simulink library "lib_cartesian_controllers"  (Simulink 9.0)
settings: Solver=ode45  StartTime=0.0  StopTime=10.0  RelTol=1e-3  EnableMultiTasking=on
undefined symbols (not defined in the file): k_D_p, k_D_r, k_p, k_P_p, k_P_r, k_r, k_t
libraries: lib_cartesian_controllers x10, lib_transformations x4
settings Model: SuppressorTable=22 serialization::archive 11 0 6 0 0 0 11 0  Creator=schappler  LastModifiedBy=schappler

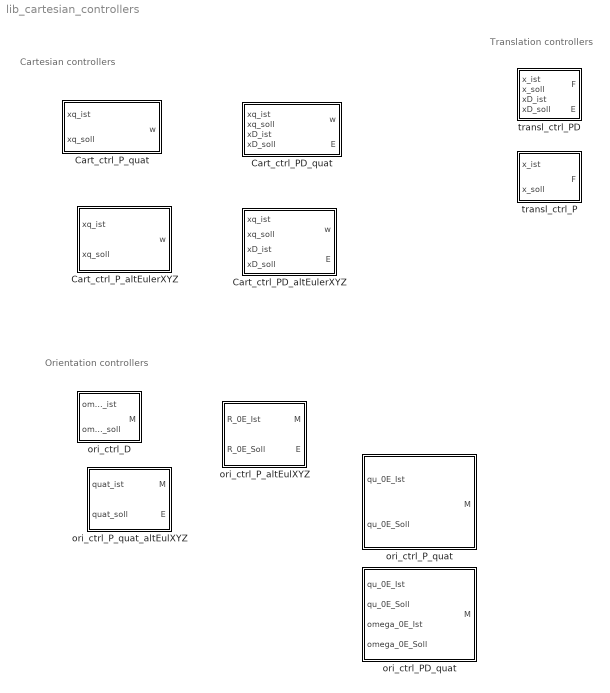
== system lib_cartesian_controllers ==
  note: Cartesian controllers
  note: Translation controllers
  note: Orientation controllers
  Cart_ctrl_PD_altEulerXYZ : Subsystem  mask{k_P_p=k_P_p, k_P_r=k_P_r, k_D_p=k_D_p, k_D_r=k_D_r}
      mask prompts: k_P_p "Translatorische Steifigkeit"; k_P_r "Rotatorische Steifigkeit"; k_D_p "Translatorische Dämpfung"; k_D_r "Rotatorische Dämpfung"
  Cart_ctrl_PD_quat : Subsystem  mask{k_P_p=k_P_p, k_P_r=k_P_r, k_D_p=k_D_p, k_D_r=k_D_r}
      mask prompts: k_P_p "Translatorische Steifigkeit"; k_P_r "Rotatorische Steifigkeit"; k_D_p "Translatorische Dämpfung"; k_D_r "Rotatorische Dämpfung"
  Cart_ctrl_P_altEulerXYZ : Subsystem  mask{k_p=k_p, k_r=k_r}
      mask prompts: k_p "Positions-Verstärkung (Steifigkeit)"; k_r "Rotations-Verstärkung (Drehsteifigkeit)"
  Cart_ctrl_P_quat : Subsystem  mask{k_t=k_t, k_r=k_r}
      mask prompts: k_t "Translatorische Steifigkeit"; k_r "Rotatorische Steifigkeit"
  ori_ctrl_D : Subsystem  mask{k=k_r}
      mask prompts: k "Proportionalverstärkung"
  ori_ctrl_PD_quat : Subsystem  mask{k_P_r=k_P_r, k_D_r=k_D_r}
      mask prompts: k_P_r "Rotatorische Steifigkeit"; k_D_r "Rotatorische Dämpfung"
  ori_ctrl_P_altEulXYZ : Subsystem  mask{k=k_r}
      mask prompts: k "Proportionalverstärkung"
  ori_ctrl_P_quat : Subsystem  mask{k_P_r=k_P_r}
      mask prompts: k_P_r "Rotatorische Steifigkeit"
  ori_ctrl_P_quat_altEulXYZ : Subsystem  mask{k_P_r=k_P_r}
      mask prompts: k_P_r "Rotatorische Steifigkeit"
  transl_ctrl_P : Subsystem  mask{k=k_t}
      mask prompts: k "Proportionalverstärkung"
  transl_ctrl_PD : Subsystem  mask{k_P_p=k_P_p, k_D_p=k_D_p}
      mask prompts: k_P_p "Proportionalverstärkung (k_P_p)"; k_D_p "Differentialverstärkung k_D_p"

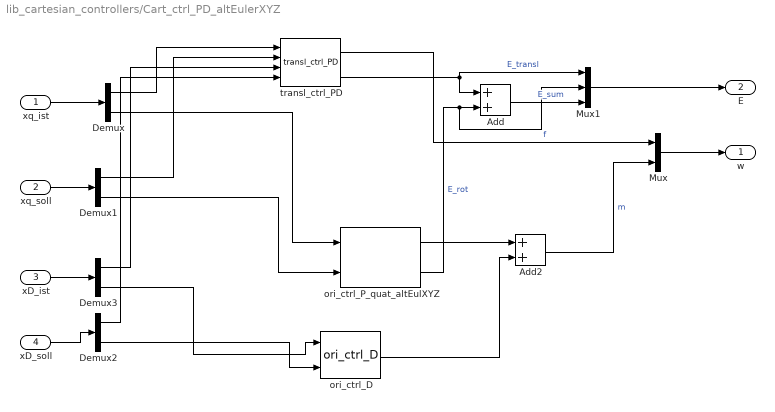
== system lib_cartesian_controllers/Cart_ctrl_PD_altEulerXYZ ==
  xq_ist : Inport  PortDimensions=7
  xq_soll : Inport  Port=2  PortDimensions=7
  xD_ist : Inport  Port=3  PortDimensions=6
  xD_soll : Inport  Port=4  PortDimensions=6
  Add : Sum
  Add2 : Sum
  Demux : Demux  Outputs=[3 4]
  Demux1 : Demux  Outputs=[3 4]
  Demux2 : Demux  Outputs=[3 3]
  Demux3 : Demux  Outputs=[3 3]
  Mux : Mux  Inputs=[3 3]
  Mux1 : Mux  Inputs=[1 1 1]
  ori_ctrl_D : lib_cartesian_controllers/ori_ctrl_D  k=k_D_r
  ori_ctrl_P_quat_altEulXYZ : lib_cartesian_controllers/ori_ctrl_P_quat_altEulXYZ  k_P_r=k_P_r
  transl_ctrl_PD : lib_cartesian_controllers/transl_ctrl_PD  k_P_p=k_P_p  k_D_p=k_D_p
  w : Outport
  E : Outport  Port=2
  wires:
  transl_ctrl_PD/1 -> Mux/1  "f"
  ori_ctrl_P_quat_altEulXYZ/1 -> Add2/1
  Demux1/1 -> transl_ctrl_PD/2
  xq_soll/1 -> Demux1/1
  Demux/1 -> transl_ctrl_PD/1
  xq_ist/1 -> Demux/1
  Demux/2 -> ori_ctrl_P_quat_altEulXYZ/1
  Demux1/2 -> ori_ctrl_P_quat_altEulXYZ/2
  xD_soll/1 -> Demux2/1
  xD_ist/1 -> Demux3/1
  Demux3/1 -> transl_ctrl_PD/3
  Demux2/1 -> transl_ctrl_PD/4
  Demux3/2 -> ori_ctrl_D/1
  Demux2/2 -> ori_ctrl_D/2
  ori_ctrl_D/1 -> Add2/2
  Mux/1 -> w/1
  Add2/1 -> Mux/2  "m"
  transl_ctrl_PD/2 -> Add/1, Mux1/1  "E_transl"
  ori_ctrl_P_quat_altEulXYZ/2 -> Mux1/2, Add/2  "E_rot"
  Mux1/1 -> E/1
  Add/1 -> Mux1/3  "E_sum"

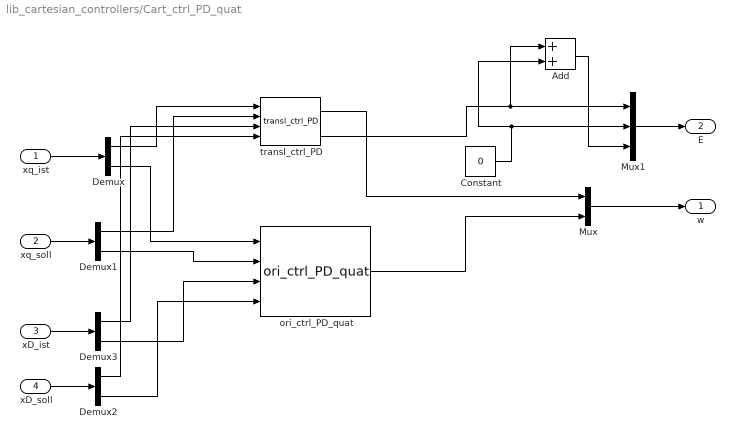
== system lib_cartesian_controllers/Cart_ctrl_PD_quat ==
  xq_ist : Inport  PortDimensions=7
  xq_soll : Inport  Port=2  PortDimensions=7
  xD_ist : Inport  Port=3  PortDimensions=6
  xD_soll : Inport  Port=4  PortDimensions=6
  Add : Sum
  Constant : Constant  Value=0
  Demux : Demux  Outputs=[3 4]
  Demux1 : Demux  Outputs=[3 4]
  Demux2 : Demux  Outputs=[3 3]
  Demux3 : Demux  Outputs=[3 3]
  Mux : Mux  Inputs=[3 3]
  Mux1 : Mux  Inputs=[1 1 1]
  ori_ctrl_PD_quat : lib_cartesian_controllers/ori_ctrl_PD_quat  k_P_r=k_P_r  k_D_r=k_D_r
  transl_ctrl_PD : lib_cartesian_controllers/transl_ctrl_PD  k_P_p=k_P_p  k_D_p=k_D_p
  w : Outport
  E : Outport  Port=2
  wires:
  Demux1/1 -> transl_ctrl_PD/2
  xq_soll/1 -> Demux1/1
  Demux/1 -> transl_ctrl_PD/1
  xq_ist/1 -> Demux/1
  Demux/2 -> ori_ctrl_PD_quat/1
  Demux1/2 -> ori_ctrl_PD_quat/2
  transl_ctrl_PD/1 -> Mux/1
  xD_soll/1 -> Demux2/1
  xD_ist/1 -> Demux3/1
  Demux3/1 -> transl_ctrl_PD/3
  Demux2/1 -> transl_ctrl_PD/4
  Demux3/2 -> ori_ctrl_PD_quat/3
  Demux2/2 -> ori_ctrl_PD_quat/4
  Mux/1 -> w/1
  ori_ctrl_PD_quat/1 -> Mux/2
  transl_ctrl_PD/2 -> Mux1/1, Add/1
  Constant/1 -> Mux1/2, Add/2
  Add/1 -> Mux1/3
  Mux1/1 -> E/1

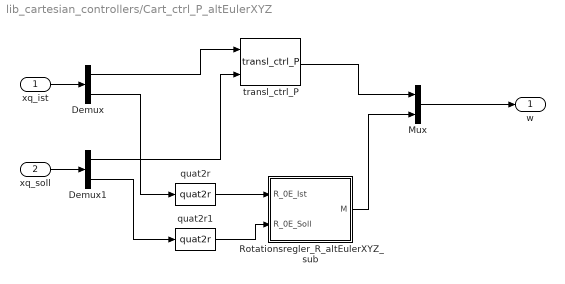
== system lib_cartesian_controllers/Cart_ctrl_P_altEulerXYZ ==
  xq_ist : Inport
  xq_soll : Inport  Port=2
  Demux : Demux  Outputs=[3 4]
  Demux1 : Demux  Outputs=[3 4]
  Mux : Mux  Inputs=[3 3]
  Rotationsregler_R_altEulerXYZ_sub : Subsystem  mask{k=k_r}
      mask prompts: k "Proportionalverstärkung"
  quat2r : lib_transformations/quat2r
  quat2r1 : lib_transformations/quat2r
  transl_ctrl_P : lib_cartesian_controllers/transl_ctrl_P  k=k_t
  w : Outport
  wires:
  transl_ctrl_P/1 -> Mux/1
  Demux1/2 -> quat2r1/1
  Demux/2 -> quat2r/1
  xq_ist/1 -> Demux/1
  Demux/1 -> transl_ctrl_P/1
  xq_soll/1 -> Demux1/1
  Demux1/1 -> transl_ctrl_P/2
  Mux/1 -> w/1
  Rotationsregler_R_altEulerXYZ_sub/1(M) -> Mux/2
  quat2r/1 -> Rotationsregler_R_altEulerXYZ_sub/1(R_0E_Ist)
  quat2r1/1 -> Rotationsregler_R_altEulerXYZ_sub/2(R_0E_Soll)

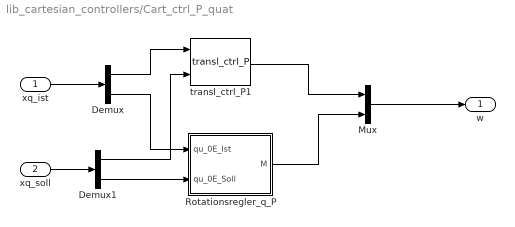
== system lib_cartesian_controllers/Cart_ctrl_P_quat ==
  xq_ist : Inport
  xq_soll : Inport  Port=2
  Demux : Demux  Outputs=[3 4]
  Demux1 : Demux  Outputs=[3 4]
  Mux : Mux  Inputs=[3 3]
  Rotationsregler_q_P : Subsystem  mask{k=k_r}
      mask prompts: k "Proportionalverstärkung"
  transl_ctrl_P1 : lib_cartesian_controllers/transl_ctrl_P  k=k_t
  w : Outport
  wires:
  transl_ctrl_P1/1 -> Mux/1
  Demux1/2 -> Rotationsregler_q_P/2(qu_0E_Soll)
  Rotationsregler_q_P/1(M) -> Mux/2
  Demux/2 -> Rotationsregler_q_P/1(qu_0E_Ist)
  xq_ist/1 -> Demux/1
  Demux/1 -> transl_ctrl_P1/1
  xq_soll/1 -> Demux1/1
  Demux1/1 -> transl_ctrl_P1/2
  Mux/1 -> w/1

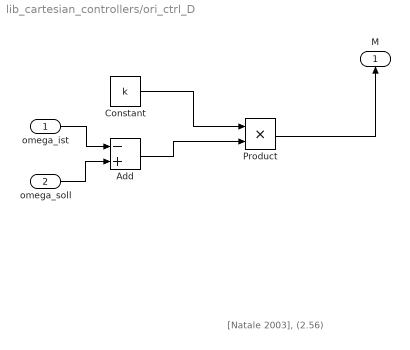
== system lib_cartesian_controllers/ori_ctrl_D ==
  note: [Natale 2003], (2.56)
  omega_ist : Inport
  omega_soll : Inport  Port=2
  Add : Sum  Inputs=-+
  Constant : Constant  Value=k
  Product : Product
  M : Outport
  wires:
  Product/1 -> M/1
  omega_ist/1 -> Add/1
  omega_soll/1 -> Add/2
  Add/1 -> Product/2
  Constant/1 -> Product/1

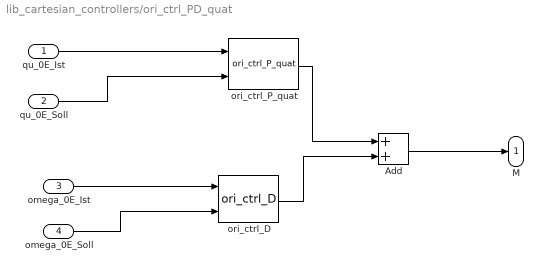
== system lib_cartesian_controllers/ori_ctrl_PD_quat ==
  qu_0E_Ist : Inport  PortDimensions=4
  qu_0E_Soll : Inport  Port=2  PortDimensions=4
  omega_0E_Ist : Inport  Port=3  PortDimensions=3
  omega_0E_Soll : Inport  Port=4  PortDimensions=3
  Add : Sum
  ori_ctrl_D : lib_cartesian_controllers/ori_ctrl_D  k=k_D_r
  ori_ctrl_P_quat : lib_cartesian_controllers/ori_ctrl_P_quat  k_P_r=k_P_r
  M : Outport  PortDimensions=3
  wires:
  qu_0E_Ist/1 -> ori_ctrl_P_quat/1
  qu_0E_Soll/1 -> ori_ctrl_P_quat/2
  Add/1 -> M/1
  omega_0E_Ist/1 -> ori_ctrl_D/1
  omega_0E_Soll/1 -> ori_ctrl_D/2
  ori_ctrl_D/1 -> Add/2
  ori_ctrl_P_quat/1 -> Add/1

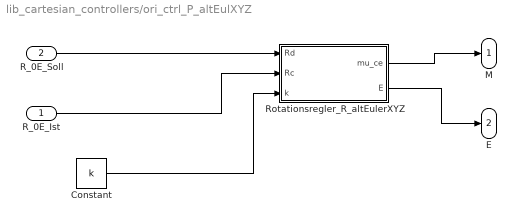
== system lib_cartesian_controllers/ori_ctrl_P_altEulXYZ ==
  R_0E_Ist : Inport  PortDimensions=[3 3]
  R_0E_Soll : Inport  Port=2  PortDimensions=[3 3]
  Constant : Constant  Value=k
  Rotationsregler_R_altEulerXYZ : MATLAB Function  TreatAsAtomicUnit=on
  M : Outport
  E : Outport  Port=2
  wires:
  Constant/1 -> Rotationsregler_R_altEulerXYZ/3(k)
  Rotationsregler_R_altEulerXYZ/1(mu_ce) -> M/1
  R_0E_Soll/1 -> Rotationsregler_R_altEulerXYZ/1(Rd)
  R_0E_Ist/1 -> Rotationsregler_R_altEulerXYZ/2(Rc)
  Rotationsregler_R_altEulerXYZ/2(E) -> E/1

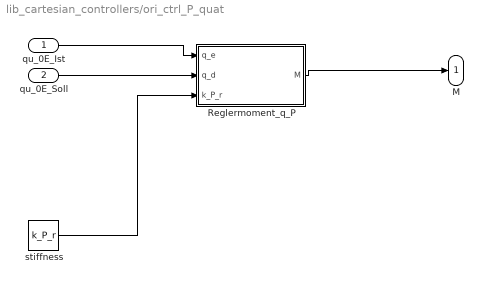
== system lib_cartesian_controllers/ori_ctrl_P_quat ==
  qu_0E_Ist : Inport  PortDimensions=4
  qu_0E_Soll : Inport  Port=2  PortDimensions=4
  Reglermoment_q_P : MATLAB Function  TreatAsAtomicUnit=on
  stiffness : Constant  Value=k_P_r
  M : Outport  PortDimensions=3
  wires:
  qu_0E_Ist/1 -> Reglermoment_q_P/1(q_e)
  qu_0E_Soll/1 -> Reglermoment_q_P/2(q_d)
  Reglermoment_q_P/1(M) -> M/1
  stiffness/1 -> Reglermoment_q_P/3(k_P_r)

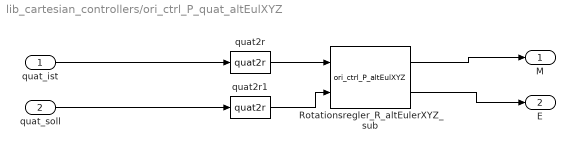
== system lib_cartesian_controllers/ori_ctrl_P_quat_altEulXYZ ==
  quat_ist : Inport
  quat_soll : Inport  Port=2
  Rotationsregler_R_altEulerXYZ_sub : lib_cartesian_controllers/ori_ctrl_P_altEulXYZ  k=k_P_r
  quat2r : lib_transformations/quat2r
  quat2r1 : lib_transformations/quat2r
  M : Outport
  E : Outport  Port=2
  wires:
  quat_soll/1 -> quat2r1/1
  quat2r/1 -> Rotationsregler_R_altEulerXYZ_sub/1
  quat_ist/1 -> quat2r/1
  Rotationsregler_R_altEulerXYZ_sub/1 -> M/1
  quat2r1/1 -> Rotationsregler_R_altEulerXYZ_sub/2
  Rotationsregler_R_altEulerXYZ_sub/2 -> E/1

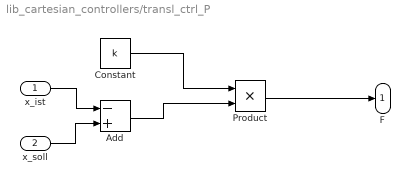
== system lib_cartesian_controllers/transl_ctrl_P ==
  x_ist : Inport
  x_soll : Inport  Port=2
  Add : Sum  Inputs=-+
  Constant : Constant  Value=k
  Product : Product
  F : Outport
  wires:
  Product/1 -> F/1
  x_ist/1 -> Add/1
  x_soll/1 -> Add/2
  Add/1 -> Product/2
  Constant/1 -> Product/1

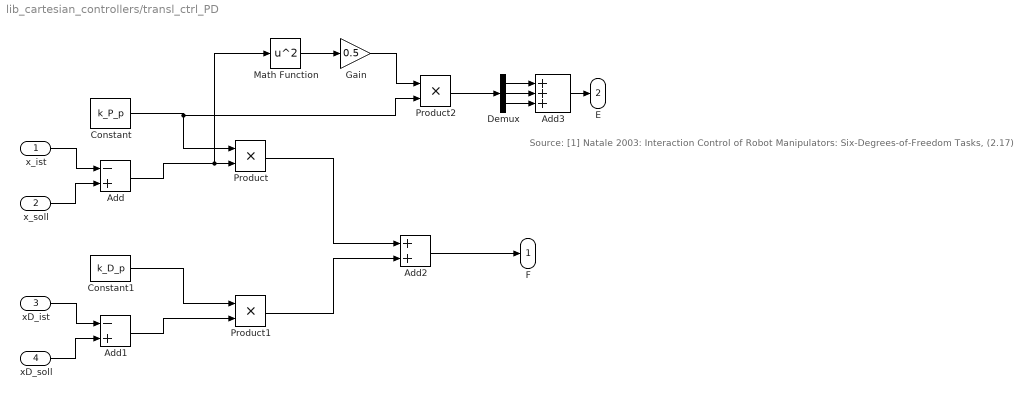
== system lib_cartesian_controllers/transl_ctrl_PD ==
  note: Source:
      | [1] Natale 2003: Interaction Control of Robot Manipulators: Six-Degrees-of-Freedom Tasks, (2.17)
  x_ist : Inport
  x_soll : Inport  Port=2
  xD_ist : Inport  Port=3
  xD_soll : Inport  Port=4
  Add : Sum  Inputs=-+
  Add1 : Sum  Inputs=-+
  Add2 : Sum
  Add3 : Sum  Inputs=+++
  Constant : Constant  Value=k_P_p
  Constant1 : Constant  Value=k_D_p
  Demux : Demux  Outputs=[1 1 1]
  Gain : Gain  Gain=0.5
  Math Function : Math  Operator=square  SaturateOnIntegerOverflow=on
  Product : Product
  Product1 : Product
  Product2 : Product
  F : Outport
  E : Outport  Port=2
  wires:
  Constant/1 -> Product2/2, Product/1
  x_soll/1 -> Add/2
  x_ist/1 -> Add/1
  Constant1/1 -> Product1/1
  Add1/1 -> Product1/2
  xD_soll/1 -> Add1/2
  xD_ist/1 -> Add1/1
  Product/1 -> Add2/1
  Product1/1 -> Add2/2
  Add2/1 -> F/1
  Add/1 -> Math Function/1, Product/2
  Math Function/1 -> Gain/1
  Product2/1 -> Demux/1
  Add3/1 -> E/1
  Demux/1 -> Add3/1
  Demux/2 -> Add3/2
  Demux/3 -> Add3/3
  Gain/1 -> Product2/1

== system lib_cartesian_controllers/Cart_ctrl_P_altEulerXYZ/Rotationsregler_R_altEulerXYZ_sub ==
  R_0E_Ist : Inport  PortDimensions=[3 3]
  R_0E_Soll : Inport  Port=2  PortDimensions=[3 3]
  Constant : Constant  Value=k
  Rotationsregler_R_altEulerXYZ : MATLAB Function  TreatAsAtomicUnit=on
  M : Outport
  wires:
  Constant/1 -> Rotationsregler_R_altEulerXYZ/3(k)
  Rotationsregler_R_altEulerXYZ/1(mu_ce) -> M/1
  R_0E_Soll/1 -> Rotationsregler_R_altEulerXYZ/1(Rd)
  R_0E_Ist/1 -> Rotationsregler_R_altEulerXYZ/2(Rc)

== system lib_cartesian_controllers/Cart_ctrl_P_quat/Rotationsregler_q_P ==
  qu_0E_Ist : Inport  PortDimensions=[4 1]
  qu_0E_Soll : Inport  Port=2  PortDimensions=[4 1]
  Constant : Constant  Value=k
  Reglermoment_q : MATLAB Function  TreatAsAtomicUnit=on
  M : Outport
  wires:
  Constant/1 -> Reglermoment_q/3(k)
  Reglermoment_q/1(M) -> M/1
  qu_0E_Soll/1 -> Reglermoment_q/1(q_d)
  qu_0E_Ist/1 -> Reglermoment_q/2(q_e)

== matlab function Cart_ctrl_P_quat/Rotationsregler_q_P/Reglermoment_q ==
  data: q_d input double; M output double; q_e input double; k input double
% Reglermoment für einen Orientierungsfehler basierend auf
% Quaternion-Darstellung

% Quellen:
% [1] Natale 2003: Interaction Control of Robot Manipulators:
% Six-Degrees-of-Freedom Tasks 

% Moritz Schappler, schappler@irt.uni-hannover.de, 2015-08
% (c) Institut für Regelungstechnik, Universität Hannover

function M = fcn(q_d, q_e, k)
%% Init
%#codegen
assert(isa(q_d,'double') && isreal(q_d) && all(size(q_d) == [4 1]), ...
  'Quaternion q_d muss [4x1] double sein.');
assert(isa(q_e,'double') && isreal(q_e) && all(size(q_e) == [4 1]), ...
  'Quaternion q_e muss [4x1] double sein.');
assert(isa(k,'double') && isreal(k) && all(size(k) == [3 1]), ...
  'Rotationssteifigkeit muss [3x1] double sein.');

%% Berechnung

% Eingangs-Quaternionen in Quaternion-Klasse umwandeln für weitere
% Operationen
Q_d = Quaternion(q_d);
Q_e = Quaternion(q_e);

% Quaternion-Orientierungsfehler: [1], (2.53)
Q_de = (Q_e.inv) * Q_d;
q_de = double(Q_de);

% Reglerausgang: [1], (2.56)
R_e = quat2r(q_e);
M = k .* (R_e * (q_de(2:4)'));

== matlab function Cart_ctrl_P_altEulerXYZ/Rotationsregler_R_altEulerXYZ_sub/Rotationsregler_R_altEulerXYZ ==
  data: Rd input double; mu_ce output double; Rc input double; k input double
% Quellen:
% [1] Natale 2003

function mu_ce = fcn(Rd, Rc, k)
%% Init
%#codegen
assert(isa(Rd,'double') && isreal(Rd) && all(size(Rd) == [3 3]), ...
  'Rotationsmatrix Rd muss [3x3] double sein.');
assert(isa(Rc,'double') && isreal(Rc) && all(size(Rc) == [3 3]), ...
  'Rotationsmatrix Rc muss [3x3] double sein.');
assert(isa(k,'double') && isreal(k) && all(size(k) == [3 1]), ...
  'Rotationssteifigkeit muss [3x3] double sein.');

%% Berechnung
% [1], (3,21)
R_cd = Rc' * Rd;

% ist xyz-euler-winkel aus Natale 2003.
phi_cd = r2rpy(R_cd);

alpha = phi_cd(1);
beta = phi_cd(2);
gamma = phi_cd(3);

T = angvelotrans_rpy(phi_cd);

mu_ce = T \ (k .* (phi_cd'));

% assert(isa(mu_ce,'double') && isreal(mu_ce) && all(size(mu_ce) == [3 1]), ...
%   'Reglermoment muss [3x1] double sein.');

== matlab function ori_ctrl_P_quat/Reglermoment_q_P ==
  data: q_e input double; q_d input double; M output double; k_P_r input double
% Reglermoment für einen Orientierungsfehler basierend auf
% Quaternion-Darstellung
% 
% Input:
% q_d
%   Soll-Orientierung (Quaternion, wxyz) des Endeffektors im Basis-KS
% q_e [3x1]
%   Ist-Orientierung (Quaternion, wxyz) des Endeffektors im Basis-KS
% k_P_r [3x1]
%   Steifigkeit (bezogen auf den Quaternionen-Imaginärteil-Winkelfehler
% 
% Output:
% M [3x1]
%   Reglermoment

% Quellen:
% [1] Natale 2003: Interaction Control of Robot Manipulators:
% Six-Degrees-of-Freedom Tasks 

% Moritz Schappler, schappler@irt.uni-hannover.de, 2015-08
% (c) Institut für Regelungstechnik, Universität Hannover

function M = fcn(q_e, q_d, k_P_r)
%% Init
%#codegen
assert(isa(q_e,'double') && isreal(q_e) && all(size(q_e) == [4 1]), ...
  'Quaternion q_e muss [4x1] double sein.');
assert(isa(q_d,'double') && isreal(q_d) && all(size(q_d) == [4 1]), ...
  'Quaternion q_d muss [4x1] double sein.');
assert(isa(k_P_r,'double') && isreal(k_P_r) && all(size(k_P_r) == [3 1]), ...
  'Rotationssteifigkeit muss [3x1] double sein.');

%% Berechnung

% Eingangs-Quaternionen in Quaternion-Klasse umwandeln für weitere
% Operationen
Q_d = Quaternion(q_d);
Q_e = Quaternion(q_e);

% Quaternion-Orientierungsfehler: [1], (2.53)
Q_de = (Q_e.inv) * Q_d;
q_de = double(Q_de);

% [1], (2.56)
R_e = quat2r(q_e);
M_P = k_P_r .* (R_e * (q_de(2:4)'));

% Reglerausgang: [1], (2.56)
M = M_P;

== matlab function ori_ctrl_P_altEulXYZ/Rotationsregler_R_altEulerXYZ ==
  data: Rd input double; mu_ce output double; Rc input double; k input double; E output double
% Kartesischer Rotationsregler basierend auf Euler-Winkeln
% 
% Eingabe:
% Rd
%   Soll-Rotation
% Rc
%   Ist-Rotation
% k
%   rotatorische Steifigkeit (in mitgedrehten Koordinaten)
% 
% Ausgabe:
% mu_ce
%   Kartesisches Moment um die gewünschte Rotation zu erreichen

% Quellen:
% [1] Natale2003: Interaction Control of Robot Manipulators:
% Six-Degrees-of-Freedom Tasks. Springer, 2003, 3 

% Moritz Schappler, schappler@irt.uni-hannover.de, 2015-09
% (C) Institut für Regelungstechnik, Universität Hannover


function [mu_ce, E] = fcn(Rd, Rc, k)
%% Init
%#codegen
assert(isa(Rd,'double') && isreal(Rd) && all(size(Rd) == [3 3]), ...
  'Rotationsmatrix Rd muss [3x3] double sein.');
assert(isa(Rc,'double') && isreal(Rc) && all(size(Rc) == [3 3]), ...
  'Rotationsmatrix Rc muss [3x3] double sein.');
assert(isa(k,'double') && isreal(k) && all(size(k) == [3 1]), ...
  'Rotationssteifigkeit muss [3x3] double sein.');

%% Berechnung
% [1], (3,21)
R_cd = Rc' * Rd;

% ist xyz-euler-winkel aus Natale 2003.
phi_cd = r2rpy(R_cd);
phi_cd = phi_cd(:);

Tw = angvelotrans_rpy(phi_cd); % [1], (2.34)
% Te = Rc*Tw; % [1], (2.31); Bereits unten eingesetzt

% Rückstellendes Moment: Federmoment in mitgedrehten Koordinaten,
% Transformation in kartesische Koordinaten mit Tw und Rotation vom KS c
% ins Welt-KS mit Rc
mu_ce = Rc * (Tw' \ (k .* phi_cd)); % [1], (2.32); Dort Transponiert-Invertiert vergessen

% Energie
E = sum(0.5 * k .* phi_cd.^2);
